simulink model "M4B11_modified_AGC_RL"  (R2025a)
settings: Solver=VariableStepAuto  StartTime=0.0  StopTime=100  RelTol=1e-3
InitFcn:
  | clear;
  | load('parameterinit.mat');
  | set_param('M4B11_modified_AGC_RL/Python2Sim1','value','[0 0]');
  | acom=100;
  | bcom=50;
  | lam=100;
  | rng('shuffle'); % 可选：先打乱 MATLAB 全局 RNG（不是必需，但说明意图）
  | seed1 = randi([1,2147483647]); % 生成 1 到 2^31-1 之间的整数
  | seed2 = randi([1,2147483647]);
values from neighbouring files (symbols this model uses):
  ACgirdinit =     [datainit.mat]    (also in parameterinit.mat)
  AVm0 = [11.3576294988 11.3576294988]    [datainit.mat]    (also in parameterinit.mat)
  commun = [1 1 1 0]    [datainit.mat]    (also in initAll.m = [1,1,1,0]; parameterinit.mat)
  DataDelay = [0  0; 0  0; 0  0; 0  0]    [datainit.mat]    (also in initAll.m = 0.0*DataDelay; parameterinit.mat)
  ESinit =     [datainit.mat]    (also in parameterinit.mat)
  fB = 50    [datainit.mat]    (also in initAll.m; parameterinit.mat)
  Geninit =     [datainit.mat]    (also in initAll.m = Generator_init(opdata,SynMach_in_gidx); parameterinit.mat)
  SgridB = 100    [datainit.mat]    (also in initAll.m = resultsac.baseMVA; parameterinit.mat)
  wB = 314.159265359    [datainit.mat]    (also in initAll.m; parameterinit.mat)
  Windinit =     [datainit.mat]    (also in parameterinit.mat)
undefined symbols (not defined in the file or in its folder): c1, c2, c3, c4, c5, c6, cp_nom, lambda_nom, P_wind_base, Pelec_base, Pnom
libraries: spsBistableLib x9, slpidlib x2, simulink_extras x2
(part 1 of 6)
settings Model: Creator=LinSiQi  LastModifiedBy=86182
settings SolverCC: AlgebraicLoopSolver=TrustRegion
settings DataIOCC: DSMLogging=off  ReturnWorkspaceOutputs=off  SignalLoggingName=logout
settings DebuggingCC: UnconnectedInputMsg=warning  UnconnectedOutputMsg=warning  UnconnectedLineMsg=warning  ArithmeticOperatorsInVariantConditions=warning
settings ModelReferenceCC: EnableRefExpFcnMdlSchedulingChecks=on
settings SFSimCC: CustomCodeUndefinedFunction=UseInterfaceOnly
settings RTWCC: GPUComputeCapability=3.5  DLArmComputeVersion=19.05
settings CodeAppCC: StateflowObjectComments=on
settings SimscapeCC: SimscapeNormalizeSystem=off

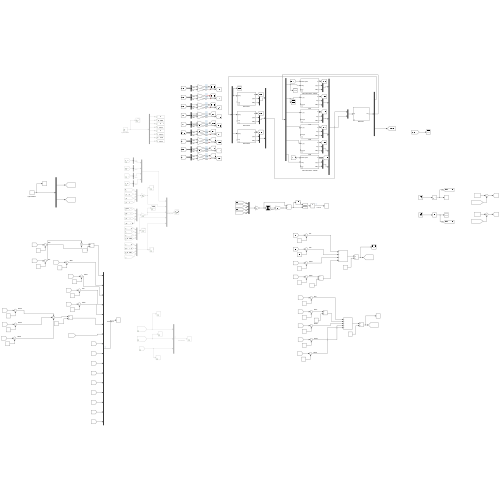
[thumbnail: Simulink's stored preview of the top-level diagram]
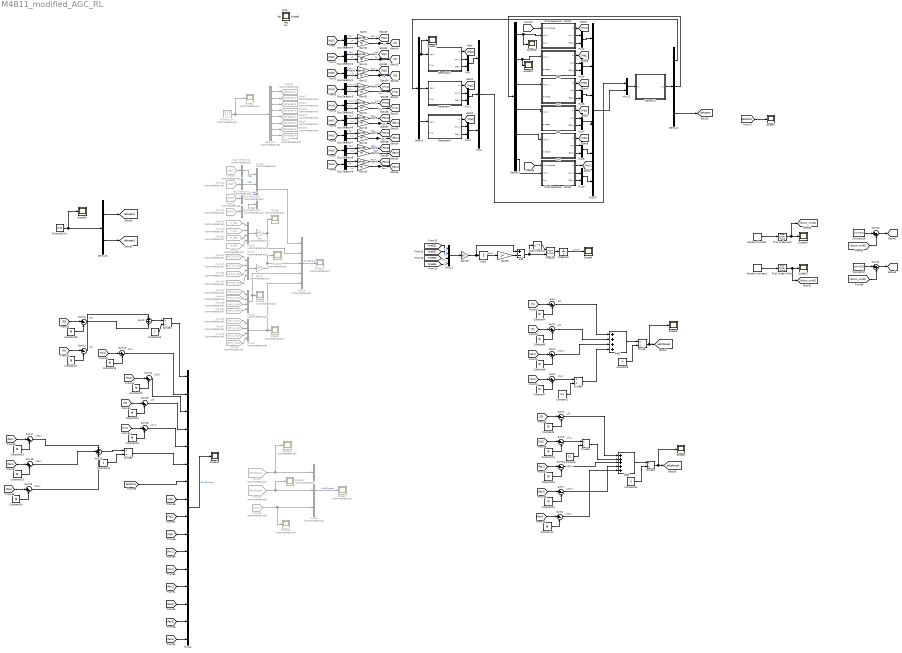
== system M4B11_modified_AGC_RL ==
  note: Δfes2
  note: Δfw2
  note: Δf3
  note: Δf1
  note: Δfes1
  note: Δfw1
  note: Δfes4
  note: Δf2
  note: Δfes3
  note: Δf1
  note: Δf2
  note: Δfw1
  note: Δfes1
  note: Δf3
  note: Δfw2
  note: Δfes4
  note: Δfes3
  note: Δfes2
  Add : Sum  Inputs=+-
  Add1 : Sum  Inputs=++++
  Add2 : Sum  Inputs=+
  Add3 : Sum  Inputs=+++++
  Bus Selector1 : BusSelector  OutputSignals=Pe,f
  Bus Selector{10..13} (4 alike) : BusSelector  Commented=on  OutputSignals=Pe
  Bus Selector2 : BusSelector  OutputSignals=Pe,f
  Bus Selector3 : BusSelector  OutputSignals=Pwind,fw
  Bus Selector4 : BusSelector  OutputSignals=Pe,f
  Bus Selector5 : BusSelector  OutputSignals=Pwind,fw
  Bus Selector{6..9} (4 alike) : BusSelector  OutputSignals=Pe,w
  Constant{4..7,9..10,12,15..25} (18 alike) : Constant  Value=fB
  Constant11 : Constant  Value=5
  Constant13 : Constant  Value=2
  Constant14 : Constant  Value=3
  Constant2 : Constant  Value=0.2
  Constant26 : Constant  Value=AVm0(1)
  Constant27 : Constant  Value=AVm0(2)
  Constant3 : Constant  Value=0.2
  Constant8 : Constant  Value=4
  Demux : Demux  Outputs=3
  Demux1 : Demux  Outputs=6
  Demux2 : Demux  Outputs=[6 12 1]
  Demux3 : Demux  Commented=on  Outputs=8
  Demux5 : Demux  Outputs=2
  Divide{,1..5} (6 alike) : Product  Inputs=*/
  ES1 : Subsystem  mask{SvscB=ESinit.SvscBi(1), SgridB=SgridB, Kppll_VSC=ESinit.Kppll(1), Kipll_VSC=ESinit.Kipll(1), Dels_hvdc=ESinit.Dels_hvdc(1), Lpr=ESinit.Lpr(1), Rpr=ESinit.Rpr(1), wB=wB, Is_xA_0=ESinit.Isx0(1), Is_yA_0=ESinit.Isy0(1), KpP_VSC_A=ESinit.KpP(1), KiP_VSC_A=ESinit.KiP(1), KpId_VSC_A=ESinit.KpId(1), KiId_VSC_A=ESinit.KiId(1), KpQ_VSC_A=ESinit.KpQ(1), KiQ_VSC_A=ESinit.KiQ(1), KpIq_VSC_A=ESinit.KpIq(1), KiIq_VSC_A=ESinit.KiIq(1), Md_A_0=ESinit.Md0(1), Mq_A_0=ESinit.Mq0(1), Nd_A_0=ESinit.Nd0(1), Nq_A_0=ESinit.Nq0(1), KIR=ESinit.Kir(1), Kdroop=ESinit.Kdroop(1), Kdistributed=ESinit.Kdistributed(1), Kdistributed_d=ESinit.Kdistributed_d(1), Kpac_VSC_A=ESinit.Kpac(1), Kiac_VSC_A=ESinit.Kiac(1), P0=ESinit.P0(1), Q0=ESinit.Q0(1), usd0=ESinit.Usd0(1)}
      mask prompts: Kppll_VSC "Kppll"; Kipll_VSC "Kipll"; KpP_VSC_A "KpP"; KiP_VSC_A "KiP"; KpId_VSC_A "KpId"; KiId_VSC_A "KiId"; KpQ_VSC_A "KpQ"; KiQ_VSC_A "KiQ"; KpIq_VSC_A "KpIq"; KiIq_VSC_A "KiIq"; Kpac_VSC_A "Kpac"; Kiac_VSC_A "Kiac"
      mask DialogControl Container48 Prompt: Base value
      mask DialogControl Container7 Prompt: PLL
      mask DialogControl Container5 Prompt: Control parameter
      mask DialogControl Container8 Prompt: inital value
      mask DialogControl Container9 Prompt: AC side
      mask DialogControl Container10 Prompt: Parameter
      mask DialogControl Container11 Prompt: Initial value
      mask DialogControl Container18 Prompt: Control parameter
      mask DialogControl Container19 Prompt: d_axis_control parameter
      mask DialogControl Container23 Prompt: d_axis_control=1
      mask DialogControl Container26 Prompt: inner current control
      mask DialogControl Container21 Prompt: q_axis_control parameter
      mask DialogControl Container29 Prompt: q_axis_control=1
      mask DialogControl Container31 Prompt: inner current control
      mask DialogControl Container22 Prompt: inital value
      mask DialogControl Container35 Prompt: outer controller
      mask DialogControl Container36 Prompt: inner control
      mask DialogControl Container27 Prompt: Inertia control
      mask DialogControl Container28 Prompt: droop control
      mask DialogControl Container300 Prompt: distributed control
      mask DialogControl Container301 Prompt: Droop distributed control
      mask DialogControl Container40 Prompt: usdq_control
      mask DialogControl Container41 Prompt: PQinitial
      mask DialogControl Container42 Prompt: usd0initial
  ES2 : Subsystem  mask{SvscB=ESinit.SvscBi(2), SgridB=SgridB, Kppll_VSC=ESinit.Kppll(2), Kipll_VSC=ESinit.Kipll(2), Dels_hvdc=ESinit.Dels_hvdc(2), Lpr=ESinit.Lpr(2), Rpr=ESinit.Rpr(2), wB=wB, Is_xA_0=ESinit.Isx0(2), Is_yA_0=ESinit.Isy0(2), KpP_VSC_A=ESinit.KpP(2), KiP_VSC_A=ESinit.KiP(2), KpId_VSC_A=ESinit.KpId(2), KiId_VSC_A=ESinit.KiId(2), KpQ_VSC_A=ESinit.KpQ(2), KiQ_VSC_A=ESinit.KiQ(2), KpIq_VSC_A=ESinit.KpIq(2), KiIq_VSC_A=ESinit.KiIq(2), Md_A_0=ESinit.Md0(2), Mq_A_0=ESinit.Mq0(2), Nd_A_0=ESinit.Nd0(2), Nq_A_0=ESinit.Nq0(2), KIR=ESinit.Kir(2), Kdroop=ESinit.Kdroop(2), Kdistributed=ESinit.Kdistributed(2), Kdistributed_d=ESinit.Kdistributed_d(2), Kpac_VSC_A=ESinit.Kpac(2), Kiac_VSC_A=ESinit.Kiac(2), P0=ESinit.P0(2), Q0=ESinit.Q0(2), usd0=ESinit.Usd0(2)}
      mask prompts: Kppll_VSC "Kppll"; Kipll_VSC "Kipll"; KpP_VSC_A "KpP"; KiP_VSC_A "KiP"; KpId_VSC_A "KpId"; KiId_VSC_A "KiId"; KpQ_VSC_A "KpQ"; KiQ_VSC_A "KiQ"; KpIq_VSC_A "KpIq"; KiIq_VSC_A "KiIq"; Kpac_VSC_A "Kpac"; Kiac_VSC_A "Kiac"
      mask DialogControl Container48 Prompt: Base value
      mask DialogControl Container7 Prompt: PLL
      mask DialogControl Container5 Prompt: Control parameter
      mask DialogControl Container8 Prompt: inital value
      mask DialogControl Container9 Prompt: AC side
      mask DialogControl Container10 Prompt: Parameter
      mask DialogControl Container11 Prompt: Initial value
      mask DialogControl Container18 Prompt: Control parameter
      mask DialogControl Container19 Prompt: d_axis_control parameter
      mask DialogControl Container23 Prompt: d_axis_control=1
      mask DialogControl Container26 Prompt: inner current control
      mask DialogControl Container21 Prompt: q_axis_control parameter
      mask DialogControl Container29 Prompt: q_axis_control=1
      mask DialogControl Container31 Prompt: inner current control
      mask DialogControl Container22 Prompt: inital value
      mask DialogControl Container35 Prompt: outer controller
      mask DialogControl Container36 Prompt: inner control
      mask DialogControl Container27 Prompt: Inertia control
      mask DialogControl Container28 Prompt: droop control
      mask DialogControl Container300 Prompt: distributed control
      mask DialogControl Container301 Prompt: Droop distributed control
      mask DialogControl Container40 Prompt: usdq_control
      mask DialogControl Container41 Prompt: PQinitial
      mask DialogControl Container42 Prompt: usd0initial
  ES3 : Subsystem  mask{SvscB=ESinit.SvscBi(3), SgridB=SgridB, Kppll_VSC=ESinit.Kppll(3), Kipll_VSC=ESinit.Kipll(3), Dels_hvdc=ESinit.Dels_hvdc(3), Lpr=ESinit.Lpr(3), Rpr=ESinit.Rpr(3), wB=wB, Is_xA_0=ESinit.Isx0(3), Is_yA_0=ESinit.Isy0(3), KpP_VSC_A=ESinit.KpP(3), KiP_VSC_A=ESinit.KiP(3), KpId_VSC_A=ESinit.KpId(3), KiId_VSC_A=ESinit.KiId(3), KpQ_VSC_A=ESinit.KpQ(3), KiQ_VSC_A=ESinit.KiQ(3), KpIq_VSC_A=ESinit.KpIq(3), KiIq_VSC_A=ESinit.KiIq(3), Md_A_0=ESinit.Md0(3), Mq_A_0=ESinit.Mq0(3), Nd_A_0=ESinit.Nd0(3), Nq_A_0=ESinit.Nq0(3), KIR=ESinit.Kir(3), Kdroop=ESinit.Kdroop(3), Kdistributed=ESinit.Kdistributed(3), Kdistributed_d=ESinit.Kdistributed_d(3), Kpac_VSC_A=ESinit.Kpac(3), Kiac_VSC_A=ESinit.Kiac(3), P0=ESinit.P0(3), Q0=ESinit.Q0(3), usd0=ESinit.Usd0(3)}
      mask prompts: Kppll_VSC "Kppll"; Kipll_VSC "Kipll"; KpP_VSC_A "KpP"; KiP_VSC_A "KiP"; KpId_VSC_A "KpId"; KiId_VSC_A "KiId"; KpQ_VSC_A "KpQ"; KiQ_VSC_A "KiQ"; KpIq_VSC_A "KpIq"; KiIq_VSC_A "KiIq"; Kpac_VSC_A "Kpac"; Kiac_VSC_A "Kiac"
      mask DialogControl Container48 Prompt: Base value
      mask DialogControl Container7 Prompt: PLL
      mask DialogControl Container5 Prompt: Control parameter
      mask DialogControl Container8 Prompt: inital value
      mask DialogControl Container9 Prompt: AC side
      mask DialogControl Container10 Prompt: Parameter
      mask DialogControl Container11 Prompt: Initial value
      mask DialogControl Container18 Prompt: Control parameter
      mask DialogControl Container19 Prompt: d_axis_control parameter
      mask DialogControl Container23 Prompt: d_axis_control=1
      mask DialogControl Container26 Prompt: inner current control
      mask DialogControl Container21 Prompt: q_axis_control parameter
      mask DialogControl Container29 Prompt: q_axis_control=1
      mask DialogControl Container31 Prompt: inner current control
      mask DialogControl Container22 Prompt: inital value
      mask DialogControl Container35 Prompt: outer controller
      mask DialogControl Container36 Prompt: inner control
      mask DialogControl Container27 Prompt: Inertia control
      mask DialogControl Container28 Prompt: droop control
      mask DialogControl Container300 Prompt: distributed control
      mask DialogControl Container301 Prompt: Droop distributed control
      mask DialogControl Container40 Prompt: usdq_control
      mask DialogControl Container41 Prompt: PQinitial
      mask DialogControl Container42 Prompt: usd0initial
  ES4 : Subsystem  mask{SvscB=ESinit.SvscBi(4), SgridB=SgridB, Kppll_VSC=ESinit.Kppll(4), Kipll_VSC=ESinit.Kipll(4), Dels_hvdc=ESinit.Dels_hvdc(4), Lpr=ESinit.Lpr(4), Rpr=ESinit.Rpr(4), wB=wB, Is_xA_0=ESinit.Isx0(4), Is_yA_0=ESinit.Isy0(4), KpP_VSC_A=ESinit.KpP(4), KiP_VSC_A=ESinit.KiP(4), KpId_VSC_A=ESinit.KpId(4), KiId_VSC_A=ESinit.KiId(4), KpQ_VSC_A=ESinit.KpQ(4), KiQ_VSC_A=ESinit.KiQ(4), KpIq_VSC_A=ESinit.KpIq(4), KiIq_VSC_A=ESinit.KiIq(4), Md_A_0=ESinit.Md0(4), Mq_A_0=ESinit.Mq0(4), Nd_A_0=ESinit.Nd0(4), Nq_A_0=ESinit.Nq0(4), KIR=ESinit.Kir(4), Kdroop=ESinit.Kdroop(4), Kdistributed=ESinit.Kdistributed(4), Kdistributed_d=ESinit.Kdistributed_d(4), Kpac_VSC_A=ESinit.Kpac(4), Kiac_VSC_A=ESinit.Kiac(4), P0=ESinit.P0(4), Q0=ESinit.Q0(4), usd0=ESinit.Usd0(4)}
      mask prompts: Kppll_VSC "Kppll"; Kipll_VSC "Kipll"; KpP_VSC_A "KpP"; KiP_VSC_A "KiP"; KpId_VSC_A "KpId"; KiId_VSC_A "KiId"; KpQ_VSC_A "KpQ"; KiQ_VSC_A "KiQ"; KpIq_VSC_A "KpIq"; KiIq_VSC_A "KiIq"; Kpac_VSC_A "Kpac"; Kiac_VSC_A "Kiac"
      mask DialogControl Container48 Prompt: Base value
      mask DialogControl Container7 Prompt: PLL
      mask DialogControl Container5 Prompt: Control parameter
      mask DialogControl Container8 Prompt: inital value
      mask DialogControl Container9 Prompt: AC side
      mask DialogControl Container10 Prompt: Parameter
      mask DialogControl Container11 Prompt: Initial value
      mask DialogControl Container18 Prompt: Control parameter
      mask DialogControl Container19 Prompt: d_axis_control parameter
      mask DialogControl Container23 Prompt: d_axis_control=1
      mask DialogControl Container26 Prompt: inner current control
      mask DialogControl Container21 Prompt: q_axis_control parameter
      mask DialogControl Container29 Prompt: q_axis_control=1
      mask DialogControl Container31 Prompt: inner current control
      mask DialogControl Container22 Prompt: inital value
      mask DialogControl Container35 Prompt: outer controller
      mask DialogControl Container36 Prompt: inner control
      mask DialogControl Container27 Prompt: Inertia control
      mask DialogControl Container28 Prompt: droop control
      mask DialogControl Container300 Prompt: distributed control
      mask DialogControl Container301 Prompt: Droop distributed control
      mask DialogControl Container40 Prompt: usdq_control
      mask DialogControl Container41 Prompt: PQinitial
      mask DialogControl Container42 Prompt: usd0initial
  First Order Hold : FirstOrderHold  ErrorTolerance=inf
  First Order Hold1 : FirstOrderHold  ErrorTolerance=inf
  From10 : From  Commented=on  GotoTag=Me2
  From11 : From  Commented=on  GotoTag=Me3
  From12 : From  Commented=on  GotoTag=Me4
  From27 : From  Commented=on  GotoTag=deltafarea1  TagVisibility=global
  From28 : From  Commented=on  GotoTag=deltafarea2  TagVisibility=global
  From29 : From  Commented=on  GotoTag=Ptie  TagVisibility=global
  From35 : From  Commented=on  GotoTag=Dess_avg4  TagVisibility=global
  From36 : From  Commented=on  GotoTag=Dess_avg3  TagVisibility=global
  From37 : From  Commented=on  GotoTag=Dess_avg2  TagVisibility=global
  From38 : From  Commented=on  GotoTag=Dess_avg1  TagVisibility=global
  From39 : From  Commented=on  GotoTag=Hess_avg3  TagVisibility=global
  From40 : From  Commented=on  GotoTag=Hess_avg2  TagVisibility=global
  From41 : From  Commented=on  GotoTag=Hess_avg1  TagVisibility=global
  From42 : From  Commented=on  GotoTag=W_ES1  TagVisibility=global
  From43 : From  Commented=on  GotoTag=ROCOF_ES1  TagVisibility=global
  From45 : From  Commented=on  GotoTag=Hess_avg4  TagVisibility=global
  From49 : From  Commented=on  GotoTag=W_ES2  TagVisibility=global
  From50 : From  Commented=on  GotoTag=ROCOF_ES2  TagVisibility=global
  From51 : From  Commented=on  GotoTag=W_ES3  TagVisibility=global
  From52 : From  Commented=on  GotoTag=ROCOF_ES3  TagVisibility=global
  From53 : From  Commented=on  GotoTag=W_ES4  TagVisibility=global
  From54 : From  Commented=on  GotoTag=ROCOF_ES4  TagVisibility=global
  From9 : From  Commented=on  GotoTag=Me1
  Gain : Gain  Commented=on  Gain=400
  Gain{1..9} (9 alike) : Gain  Gain=SgridB
  Gain{10..16,20..21} (9 alike) : Gain  Gain=fB
  Gain17 : Gain  Commented=on  Gain=200
  Gain18 : Gain  Gain=1/4
  Gain19 : Gain  Gain=50
  Generator1 : Subsystem  mask{wB=wB, SgenB=Geninit.SgenB(1), SgridB=SgridB, Xq=Geninit.Xq(1), Xq1=Geninit.Xq1(1), Xq11=Geninit.Xq11(1), Tq0=Geninit.Tq0(1), Tq10=Geninit.Tq10(1), Eq10=Geninit.Eq1(1), Eq110=Geninit.Eq11(1), Xd=Geninit.Xd(1), Xd1=Geninit.Xd1(1), Xd11=Geninit.Xd11(1), Td0=Geninit.Td0(1), Td10=Geninit.Td10(1), Ed10=Geninit.Ed1(1), Ed110=Geninit.Ed11(1), H=Geninit.Tj(1), D=Geninit.D(1), delta0=Geninit.Delta(1), w0=1, Pm0=Geninit.Pm0(1), Ka=Geninit.Ka(1), Tb=Geninit.Tb(1), Tc=Geninit.Tc(1), Efmin=Geninit.Efmin(1), Efmax=Geninit.Efmax(1), Vref=Geninit.Vref(1), Ef10=Geninit.Vf1(1), S_PSS=Geninit.EnablePSS(1), Kpss=Geninit.kpss(1), Tw_P=Geninit.Tw_P(1), T1_P=Geninit.T1_P(1), T2_P=Geninit.T2_P(1), T3_P=Geninit.T3_P(1), T4_P=Geninit.T4_P(1), Upmax=Geninit.Upmax(1), Upmin=Geninit.Upmin(1), S_Gov=Geninit.Enablegov(1), R=Geninit.R_G(1), Ts_G=Geninit.Ts_G(1), Tc_G=Geninit.Tc_G(1), T3_G=Geninit.T3_G(1), T4_G=Geninit.T4_G(1), T5_G=Geninit.T5_G(1), dPmax=Geninit.dPmax(1), dPmin=Geninit.dPmin(1)}
      mask prompts: S_PSS "Enable PSS"; Tw_P "Tw"; T1_P "T1"; T2_P "T2"; T3_P "T3"; T4_P "T4"; S_Gov "Enable Governor"; Ts_G "Ts"; Tc_G "Tc"; T3_G "T3"; T4_G "T4"; T5_G "T5"
      mask help: This is a six-order synchronous generator with exciter system, governor and PSS.
      mask DialogControl Container6 Prompt: Machine parameter
      mask DialogControl Container25 Prompt: Base value
      mask DialogControl Container3 Prompt: q axis parameter
      mask DialogControl ParameterGroupVar Prompt: d axis parameter
      mask DialogControl Container4 Prompt: machine parameter
      mask DialogControl Container12 Prompt: Excitation System parameter
      mask DialogControl Container22 Prompt: parameter
      mask DialogControl Container23 Prompt: inital value
      mask DialogControl Container10 Prompt: PSS parameter
      mask DialogControl Container13 Prompt: Governor parameter
  Generator2 : Subsystem  mask{wB=wB, SgenB=Geninit.SgenB(2), SgridB=SgridB, Xq=Geninit.Xq(2), Xq1=Geninit.Xq1(2), Xq11=Geninit.Xq11(2), Tq0=Geninit.Tq0(2), Tq10=Geninit.Tq10(2), Eq10=Geninit.Eq1(2), Eq110=Geninit.Eq11(2), Xd=Geninit.Xd(2), Xd1=Geninit.Xd1(2), Xd11=Geninit.Xd11(2), Td0=Geninit.Td0(2), Td10=Geninit.Td10(2), Ed10=Geninit.Ed1(2), Ed110=Geninit.Ed11(2), H=Geninit.Tj(2), D=Geninit.D(2), delta0=Geninit.Delta(2), w0=1, Pm0=Geninit.Pm0(2), Ka=Geninit.Ka(2), Tb=Geninit.Tb(2), Tc=Geninit.Tc(2), Efmin=Geninit.Efmin(2), Efmax=Geninit.Efmax(2), Vref=Geninit.Vref(2), Ef10=Geninit.Vf1(2), S_PSS=Geninit.EnablePSS(2), Kpss=Geninit.kpss(2), Tw_P=Geninit.Tw_P(2), T1_P=Geninit.T1_P(2), T2_P=Geninit.T2_P(2), T3_P=Geninit.T3_P(2), T4_P=Geninit.T4_P(2), Upmax=Geninit.Upmax(2), Upmin=Geninit.Upmin(2), S_Gov=Geninit.Enablegov(2), R=Geninit.R_G(2), Ts_G=Geninit.Ts_G(2), Tc_G=Geninit.Tc_G(2), T3_G=Geninit.T3_G(2), T4_G=Geninit.T4_G(2), T5_G=Geninit.T5_G(2), dPmax=Geninit.dPmax(2), dPmin=Geninit.dPmin(2)}
      mask prompts: S_PSS "Enable PSS"; Tw_P "Tw"; T1_P "T1"; T2_P "T2"; T3_P "T3"; T4_P "T4"; S_Gov "Enable Governor"; Ts_G "Ts"; Tc_G "Tc"; T3_G "T3"; T4_G "T4"; T5_G "T5"
      mask help: This is a six-order synchronous generator with exciter system, governor and PSS.
      mask DialogControl Container6 Prompt: Machine parameter
      mask DialogControl Container25 Prompt: Base value
      mask DialogControl Container3 Prompt: q axis parameter
      mask DialogControl ParameterGroupVar Prompt: d axis parameter
      mask DialogControl Container4 Prompt: machine parameter
      mask DialogControl Container12 Prompt: Excitation System parameter
      mask DialogControl Container22 Prompt: parameter
      mask DialogControl Container23 Prompt: inital value
      mask DialogControl Container10 Prompt: PSS parameter
      mask DialogControl Container13 Prompt: Governor parameter
  Generator3 : Subsystem  mask{wB=wB, SgenB=Geninit.SgenB(3), SgridB=SgridB, Xq=Geninit.Xq(3), Xq1=Geninit.Xq1(3), Xq11=Geninit.Xq11(3), Tq0=Geninit.Tq0(3), Tq10=Geninit.Tq10(3), Eq10=Geninit.Eq1(3), Eq110=Geninit.Eq11(3), Xd=Geninit.Xd(3), Xd1=Geninit.Xd1(3), Xd11=Geninit.Xd11(3), Td0=Geninit.Td0(3), Td10=Geninit.Td10(3), Ed10=Geninit.Ed1(3), Ed110=Geninit.Ed11(3), H=Geninit.Tj(3), D=Geninit.D(3), delta0=Geninit.Delta(3), w0=1, Pm0=Geninit.Pm0(3), Ka=Geninit.Ka(3), Tb=Geninit.Tb(3), Tc=Geninit.Tc(3), Efmin=Geninit.Efmin(3), Efmax=Geninit.Efmax(3), Vref=Geninit.Vref(3), Ef10=Geninit.Vf1(3), S_PSS=Geninit.EnablePSS(3), Kpss=Geninit.kpss(3), Tw_P=Geninit.Tw_P(3), T1_P=Geninit.T1_P(3), T2_P=Geninit.T2_P(3), T3_P=Geninit.T3_P(3), T4_P=Geninit.T4_P(3), Upmax=Geninit.Upmax(3), Upmin=Geninit.Upmin(3), S_Gov=Geninit.Enablegov(3), R=Geninit.R_G(3), Ts_G=Geninit.Ts_G(3), Tc_G=Geninit.Tc_G(3), T3_G=Geninit.T3_G(3), T4_G=Geninit.T4_G(3), T5_G=Geninit.T5_G(3), dPmax=Geninit.dPmax(3), dPmin=Geninit.dPmin(3)}
      mask prompts: S_PSS "Enable PSS"; Tw_P "Tw"; T1_P "T1"; T2_P "T2"; T3_P "T3"; T4_P "T4"; S_Gov "Enable Governor"; Ts_G "Ts"; Tc_G "Tc"; T3_G "T3"; T4_G "T4"; T5_G "T5"
      mask help: This is a six-order synchronous generator with exciter system, governor and PSS.
      mask DialogControl Container6 Prompt: Machine parameter
      mask DialogControl Container25 Prompt: Base value
      mask DialogControl Container3 Prompt: q axis parameter
      mask DialogControl ParameterGroupVar Prompt: d axis parameter
      mask DialogControl Container4 Prompt: machine parameter
      mask DialogControl Container12 Prompt: Excitation System parameter
      mask DialogControl Container22 Prompt: parameter
      mask DialogControl Container23 Prompt: inital value
      mask DialogControl Container10 Prompt: PSS parameter
      mask DialogControl Container13 Prompt: Governor parameter
  Goto10 : Goto  Commented=on  GotoTag=deltaDess1  TagVisibility=global
  Goto11 : Goto  Commented=on  GotoTag=deltaHess2  TagVisibility=global
  Goto12 : Goto  Commented=on  GotoTag=deltaHess1  TagVisibility=global
  Goto16 : Goto  Commented=on  GotoTag=deltaHess4  TagVisibility=global
  Goto17 : Goto  Commented=on  GotoTag=deltaHess3  TagVisibility=global
  Goto18 : Goto  Commented=on  GotoTag=deltaDess4  TagVisibility=global
  Goto19 : Goto  Commented=on  GotoTag=deltaDess3  TagVisibility=global
  Goto9 : Goto  Commented=on  GotoTag=deltaDess2  TagVisibility=global
  Integrator : Integrator
  Math Function : Math  Operator=transpose
  Mux{,1..3,5..9,11} (10 alike) : Mux  Inputs=2
  Mux10 : Mux  Inputs=6
  Mux{12,20..23} (5 alike) : Mux  Commented=on
  Mux13 : Mux
  Mux14 : Mux  Inputs=16
  Mux19 : Mux  Commented=on  Inputs=3
  Mux24 : Mux  Commented=on  Inputs=5
  Mux4 : Mux  Inputs=3
  Network1 : Subsystem  mask{busdata=ACgirdinit.busdata{1}, linedata=ACgirdinit.linedata{1}, VSS0=ACgirdinit.VSS0{1}, LINE=ACgirdinit.fline{1}, fbus=ACgirdinit.FBUS(1), ng=ACgirdinit.ng{1}, Currentin_idx=ACgirdinit.Currentin_idx{1}, amp=ACgirdinit.amp}
  Product : Product  Multiplication=Matrix(*)
  Python2Sim : Constant  Commented=on  Value=[0 0 0 0 0 0 0 0]
  Python2Sim1 : Constant  Value=[0 0]
  Random Number : RandomNumber  Variance=0  Seed=seed1  SampleTime=0.2
  Random Number1 : RandomNumber  Variance=0  Seed=seed2  SampleTime=0.2
  Scope{,1..4,10..12,14,16} (10 alike) : Scope  Commented=on
      Scope settings: ActiveDisplayYMinimum=-0.00781  ActiveDisplayYMaximum=0.06976  DataLoggingVariableName=ScopeData7
      Scope1 settings: ActiveDisplayYMinimum=-1  ActiveDisplayYMaximum=1  DataLoggingVariableName=ScopeData5
      Scope10 settings: ActiveDisplayYMinimum=-0.00781  ActiveDisplayYMaximum=0.06976
      Scope11 settings: ActiveDisplayYMinimum=-0.65989  ActiveDisplayYMaximum=0.16966  DataLoggingVariableName=ScopeData2
      Scope12 settings: ActiveDisplayYMinimum=-2.31076  ActiveDisplayYMaximum=1.65079  DataLoggingVariableName=ScopeData3
      Scope14 settings: ActiveDisplayYMinimum=-1  ActiveDisplayYMaximum=1  DataLoggingVariableName=ScopeData5
      Scope16 settings: ActiveDisplayYMinimum=-0.65989  ActiveDisplayYMaximum=0.16966  DataLoggingVariableName=ScopeData11
      Scope2 settings: ActiveDisplayYMinimum=-2.31076  ActiveDisplayYMaximum=1.65079  DataLoggingVariableName=ScopeData8
      Scope3 settings: ActiveDisplayYMinimum=-0.04265  ActiveDisplayYMaximum=0.38387  DataLoggingVariableName=ScopeData9
      Scope4 settings: ActiveDisplayYMinimum=-1  ActiveDisplayYMaximum=1  DataLoggingVariableName=ScopeData10
  Scope{5..9,13,15,17..21} (12 alike) : Scope
      Scope13 settings: ActiveDisplayYMinimum=-20.35289  ActiveDisplayYMaximum=182.95724
      Scope15 settings: ActiveDisplayYMinimum=-1  ActiveDisplayYMaximum=1
      Scope17 settings: DataLoggingVariableName=ScopeData16
      Scope18 settings: DataLoggingVariableName=ScopeData17
      Scope19 settings: ActiveDisplayYMinimum=-1  ActiveDisplayYMaximum=1  DataLoggingVariableName=ScopeData23
      Scope20 settings: ActiveDisplayYMinimum=-2.2489543876139111  ActiveDisplayYMaximum=3.3539392148111777  DataLoggingVariableName=ScopeData18
      Scope21 settings: ActiveDisplayYMinimum=-3.4452863653493173  ActiveDisplayYMaximum=3.6369803120359561  DataLoggingVariableName=ScopeData19
      Scope5 settings: ActiveDisplayYMinimum=-6E-10  ActiveDisplayYMaximum=5.2E-9
      Scope7 settings: ActiveDisplayYMinimum=-0.37863  ActiveDisplayYMaximum=3.18886  DataLoggingVariableName=ScopeData2
      Scope8 settings: ActiveDisplayYMinimum=-1.41249  ActiveDisplayYMaximum=12.71242  DataLoggingVariableName=ScopeData2
      Scope9 settings: ActiveDisplayYMinimum=-1.97687  ActiveDisplayYMaximum=17.79187  DataLoggingVariableName=ScopeData3
      Scope6 settings: ActiveDisplayYMinimum=49.70428094700177  ActiveDisplayYMaximum=50.075704699720347
  Sum{,1..8,11..19} (18 alike) : Sum  Inputs=|+-
  Sum10 : Sum  Inputs=+++
  Sum20 : Sum  Inputs=|++
  Sum21 : Sum  Inputs=|++
  Sum9 : Sum
  Wind Generator - DFIG1 : Subsystem  mask{NN=Windinit.NN(1), SwgBi=Windinit.SwgBi(1), SmecBi=100, SgridB=SgridB, Atheta=Windinit.Atheta(1), Kppll=Windinit.Kppll_wind(1), Kipll=Windinit.Kipll_wind(1), pitch=[500 45 2], Srotors=1.3, H=Windinit.H(1), Wr0=Windinit.Wr0(1), Xa=Windinit.Xa(1), Xa1=Windinit.Xa1(1), Lm=Windinit.Lm(1), Lr=Windinit.Lr(1), Rs=Windinit.Rs(1), Ls=Windinit.Ls(1), Ta0=Windinit.Ta0(1), NPf=Windinit.NPf(1), Za=Windinit.Za{1}, Ex0=Windinit.Ex_ref(1), Ey0=Windinit.Ey_ref(1), wB=wB, KpP_rw=Windinit.KpP_rw(1), KiP_rw=Windinit.KiP_rw(1), KpId_rw=Windinit.KpId_rw(1), KiId_rw=Windinit.KiId_rw(1), KpQ_rw=Windinit.KpQ_rw(1), KiQ_rw=Windinit.KiQ_rw(1), KpIq_rw=Windinit.KpIq_rw(1), KiIq_rw=Windinit.KiIq_rw(1), Ird_ref=Windinit.Ird_ref(1), Irq_ref=Windinit.Irq_ref(1), Qs0=Windinit.Qs0(1), KpDC_gw=Windinit.KpDC_gw(1), KiDC_gw=Windinit.KiDC_gw(1), KpId_gw=Windinit.KpId_gw(1), KiId_gw=Windinit.KiId_gw(1), KpIq_gw=Windinit.KpIq_gw(1), KiIq_gw=Windinit.KiIq_gw(1), Vdc_w=Windinit.Vdc_w(1), Icd_ref=Windinit.Icd_ref(1), Icq_ref=Windinit.Icq_ref(1), Vcd_ref=Windinit.Vcd_ref(1), Vcq_ref=Windinit.Vcq_ref(1), Lg=Windinit.Lg(1), Rg=Windinit.Rg(1), Icx0=Windinit.Icx0(1), Icy0=Windinit.Icy0(1), C_w=Windinit.C_w(1), Vdc0=Windinit.Vdc0(1)}
      mask prompts: pitch "pitch_gain，pitch_max，pitch_rate"; Srotors "Start Rotor Speed"; Ex0 "Ex"; Ey0 "Ey"
      mask init:
      | pitch_gain=pitch(1);
      | pitch_max=pitch(2);
      | pitch_rate=pitch(3);
      | 
      | %该风机模型的基准容量
      | 
      | SwgeqB=SwgBi.*NN;
      mask DialogControl Container4 Prompt: PLL/Wind turbine
      mask DialogControl Container31 Prompt: Base value
      mask DialogControl Container23 Prompt: PLL
      mask DialogControl Container6 Prompt: inital value
      mask DialogControl Container5 Prompt: PI parameter
      mask DialogControl Container24 Prompt: Wind turbine
      mask DialogControl Container25 Prompt: pitch control
      mask DialogControl Container7 Prompt: Machine parameter
      mask DialogControl Container8 Prompt: Rotor
      mask DialogControl Container9 Prompt: Machine
      mask DialogControl Container10 Prompt: parameter
      mask DialogControl Container11 Prompt: inital value
      mask DialogControl Container12 Prompt: Rotor side control
      mask DialogControl Container13 Prompt: Control parameter
      mask DialogControl Container14 Prompt: Initial value
      mask DialogControl Container15 Prompt: reactive power
      mask DialogControl Container16 Prompt: Grid side control
      mask DialogControl Container17 Prompt: parameter
      mask DialogControl Container18 Prompt: reference
      mask DialogControl Container19 Prompt: inital value
      mask DialogControl Container20 Prompt: converter function
      mask DialogControl Container21 Prompt: inital value
      mask DialogControl Container22 Prompt: DC function
  Wind Generator - DFIG2 : Subsystem  mask{NN=Windinit.NN(2), SwgBi=Windinit.SwgBi(2), SmecBi=100, SgridB=SgridB, Atheta=Windinit.Atheta(2), Kppll=Windinit.Kppll_wind(2), Kipll=Windinit.Kipll_wind(2), pitch=[500 45 2], Srotors=1.3, H=Windinit.H(2), Wr0=Windinit.Wr0(2), Xa=Windinit.Xa(2), Xa1=Windinit.Xa1(2), Lm=Windinit.Lm(2), Lr=Windinit.Lr(2), Rs=Windinit.Rs(2), Ls=Windinit.Ls(2), Ta0=Windinit.Ta0(2), NPf=Windinit.NPf(2), Za=Windinit.Za{2}, Ex0=Windinit.Ex_ref(2), Ey0=Windinit.Ey_ref(2), wB=wB, KpP_rw=Windinit.KpP_rw(2), KiP_rw=Windinit.KiP_rw(2), KpId_rw=Windinit.KpId_rw(2), KiId_rw=Windinit.KiId_rw(2), KpQ_rw=Windinit.KpQ_rw(2), KiQ_rw=Windinit.KiQ_rw(2), KpIq_rw=Windinit.KpIq_rw(2), KiIq_rw=Windinit.KiIq_rw(2), Ird_ref=Windinit.Ird_ref(2), Irq_ref=Windinit.Irq_ref(2), Qs0=Windinit.Qs0(2), KpDC_gw=Windinit.KpDC_gw(2), KiDC_gw=Windinit.KiDC_gw(2), KpId_gw=Windinit.KpId_gw(2), KiId_gw=Windinit.KiId_gw(2), KpIq_gw=Windinit.KpIq_gw(2), KiIq_gw=Windinit.KiIq_gw(2), Vdc_w=Windinit.Vdc_w(2), Icd_ref=Windinit.Icd_ref(2), Icq_ref=Windinit.Icq_ref(2), Vcd_ref=Windinit.Vcd_ref(2), Vcq_ref=Windinit.Vcq_ref(2), Lg=Windinit.Lg(2), Rg=Windinit.Rg(2), Icx0=Windinit.Icx0(2), Icy0=Windinit.Icy0(2), C_w=Windinit.C_w(2), Vdc0=Windinit.Vdc0(2)}
      mask prompts: pitch "pitch_gain，pitch_max，pitch_rate"; Srotors "Start Rotor Speed"; Ex0 "Ex"; Ey0 "Ey"
      mask init:
      | pitch_gain=pitch(1);
      | pitch_max=pitch(2);
      | pitch_rate=pitch(3);
      | 
      | %该风机模型的基准容量
      | 
      | SwgeqB=SwgBi.*NN;
      mask DialogControl Container4 Prompt: PLL/Wind turbine
      mask DialogControl Container31 Prompt: Base value
      mask DialogControl Container23 Prompt: PLL
      mask DialogControl Container6 Prompt: inital value
      mask DialogControl Container5 Prompt: PI parameter
      mask DialogControl Container24 Prompt: Wind turbine
      mask DialogControl Container25 Prompt: pitch control
      mask DialogControl Container7 Prompt: Machine parameter
      mask DialogControl Container8 Prompt: Rotor
      mask DialogControl Container9 Prompt: Machine
      mask DialogControl Container10 Prompt: parameter
      mask DialogControl Container11 Prompt: inital value
      mask DialogControl Container12 Prompt: Rotor side control
      mask DialogControl Container13 Prompt: Control parameter
      mask DialogControl Container14 Prompt: Initial value
      mask DialogControl Container15 Prompt: reactive power
      mask DialogControl Container16 Prompt: Grid side control
      mask DialogControl Container17 Prompt: parameter
      mask DialogControl Container18 Prompt: reference
      mask DialogControl Container19 Prompt: inital value
      mask DialogControl Container20 Prompt: converter function
      mask DialogControl Container21 Prompt: inital value
      mask DialogControl Container22 Prompt: DC function
  Pes : Scope
      settings: ActiveDisplayYMinimum=-12.906510922619532  ActiveDisplayYMaximum=250.25539940171976  DataLoggingVariableName=ScopeData4
  Pg : Scope
      settings: ActiveDisplayYMinimum=559.168910466539  ActiveDisplayYMaximum=845.17141516748893
  Pw : Scope
      settings: ActiveDisplayYMinimum=14.4539  ActiveDisplayYMaximum=655.57738  DataLoggingVariableName=ScopeData3
  fes : Scope
      settings: ActiveDisplayYMinimum=49.6543119958632  ActiveDisplayYMaximum=50.103977263973036  DataLoggingVariableName=ScopeData6
  fg : Scope
      settings: ActiveDisplayYMinimum=49.808347560980451  ActiveDisplayYMaximum=50.045408030054375  DataLoggingVariableName=ScopeData2
  tag scope: deltaPtie=global, deltafarea1=global, deltafarea2=global, deltapes1=global, deltapes3=global
  wires:
  Mux/1 -> Mux4/1
  Generator2/2(Igxy1) -> Mux1/1
  Generator3/2(Igxy1) -> Mux2/1
  Generator1/2(Igxy1) -> Mux/1
  Generator2/3(GBxy) -> Mux1/2
  Mux1/1 -> Mux4/2
  Mux2/1 -> Mux4/3
  Generator1/3(GBxy) -> Mux/2
  Generator3/3(GBxy) -> Mux2/2
  Demux/2 -> Generator2/1(Vgxy)
  Demux/3 -> Generator3/1(Vgxy)
  Demux1/1 -> Scope18/1, Wind Generator - DFIG1/2(Vsxy)
  Demux1/2 -> Scope19/1, ES1/1(us_xy)
  Demux1/3 -> ES2/1(us_xy)
  Demux1/4 -> ES3/1(us_xy)
  Demux1/5 -> ES4/1(us_xy)
  Demux1/6 -> Wind Generator - DFIG2/2(Vsxy)
  Wind Generator - DFIG1/3(GBxy) -> Mux3/2
  Mux3/1 -> Mux10/1
  Wind Generator - DFIG1/2(Igxy1) -> Mux3/1
  ES1/3(GBxy) -> Mux5/2
  Mux5/1 -> Mux10/2
  ES1/2(isxy) -> Mux5/1
  ES2/3(GBxy) -> Mux6/2
  Mux6/1 -> Mux10/3
  ES2/2(isxy) -> Mux6/1
  ES3/3(GBxy) -> Mux7/2
  Mux7/1 -> Mux10/4
  ES3/2(isxy) -> Mux7/1
  ES4/3(GBxy) -> Mux8/2
  Mux8/1 -> Mux10/5
  ES4/2(isxy) -> Mux8/1
  Wind Generator - DFIG2/3(GBxy) -> Mux9/2
  Mux9/1 -> Mux10/6
  Wind Generator - DFIG2/2(Igxy1) -> Mux9/1
  Network1/1(Vxy) -> Demux2/1
  Demux2/1 -> Demux/1
  Demux2/2 -> Demux1/1
  Mux11/1 -> Network1/1(Ixy)
  Mux4/1 -> Mux11/1
  Mux10/1 -> Mux11/2
  Generator1/1(m) -> [Mg1]
  Generator2/1(m) -> [Mg2]
  Generator3/1(m) -> [Mg3]
  Wind Generator - DFIG1/1(m) -> [Mw1]
  Wind Generator - DFIG2/1(m) -> [Mw2]
  ES2/1(m) -> [Me2]
  ES1/1(m) -> [Me1]
  ES3/1(m) -> [Me3]
  ES4/1(m) -> [Me4]
  [Mg1] -> Bus Selector4/1
  Bus Selector4/1 -> Gain6/1  "<Pe>"
  Bus Selector1/1 -> Gain1/1  "<Pe>"
  [Mg2] -> Bus Selector1/1
  Bus Selector1/2 -> Gain11/1  "<f>"
  Bus Selector2/1 -> Gain2/1  "<Pe>"
  [Mg3] -> Bus Selector2/1
  Bus Selector2/2 -> Gain12/1  "<f>"
  [Mw1] -> Bus Selector3/1
  Bus Selector3/1 -> Gain3/1  "<Pwind>"
  [Mw2] -> Bus Selector5/1
  Bus Selector5/1 -> Gain4/1  "<Pwind>"
  [Me1] -> Bus Selector6/1
  Bus Selector6/1 -> Gain5/1  "<Pe>"
  Gain6/1 -> [Pg1]  "Pg1"
  Gain1/1 -> ?  "Pg2"
  Gain2/1 -> [Pg3]  "Pg3"
  Gain3/1 -> [Pw1]  "Pw1"
  Gain4/1 -> [Pw2]  "Pw2"
  Gain5/1 -> [Pes1]  "Pes1"
  Gain7/1 -> [Pes2]  "Pes2"
  Bus Selector7/1 -> Gain7/1  "<Pe>"
  [Me2] -> Bus Selector7/1
  [Me3] -> Bus Selector8/1
  Bus Selector8/1 -> Gain8/1  "<Pe>"
  Gain8/1 -> [Pes3]  "Pes3"
  [Me4] -> Bus Selector9/1
  Bus Selector9/1 -> Gain9/1  "<Pe>"
  Gain9/1 -> [Pes4]  "Pes4"
  Gain10/1 -> [f1]  "f1"
  Bus Selector4/2 -> Gain10/1  "<f>"
  Gain11/1 -> [f2]  "f2"
  Gain12/1 -> [f3]  "f3"
  Demux3/4 -> Goto16/1
  Demux3/5 -> Goto10/1
  Demux3/6 -> Goto9/1
  Demux3/7 -> Goto19/1
  Python2Sim/1 -> Scope1/1, Demux3/1
  Demux3/2 -> Goto11/1
  Demux3/3 -> Goto17/1
  Demux3/1 -> Goto12/1
  Demux3/8 -> Goto18/1
  Bus Selector6/2 -> Gain13/1  "<w>"
  Bus Selector7/2 -> Gain14/1  "<w>"
  Bus Selector8/2 -> Gain15/1  "<w>"
  Bus Selector9/2 -> Gain16/1  "<w>"
  Gain13/1 -> [fes1]  "fes1"
  Gain14/1 -> [fes2]  "fes2"
  Gain15/1 -> [fes3]  "fes3"
  Gain16/1 -> [fes4]  "fes4"
  From9/1 -> Bus Selector10/1
  From10/1 -> Bus Selector11/1
  From11/1 -> Bus Selector12/1
  From12/1 -> Bus Selector13/1
  Bus Selector12/1 -> Mux12/3  "<Pe>"
  Bus Selector13/1 -> Mux12/4  "<Pe>"
  Bus Selector11/1 -> Mux12/2  "<Pe>"
  Bus Selector10/1 -> Mux12/1  "<Pe>"
  From42/1 -> Mux20/1
  From51/1 -> Mux20/3
  From53/1 -> Mux20/4
  From49/1 -> Mux20/2
  Gain/1 -> Scope/1, Mux24/2
  Mux20/1 -> Gain/1
  From52/1 -> Mux21/3
  From50/1 -> Mux21/2
  From54/1 -> Mux21/4
  From43/1 -> Mux21/1
  Gain17/1 -> Scope2/1, Mux24/3
  Mux21/1 -> Gain17/1
  Mux23/1 -> Mux24/4, Scope3/1
  From45/1 -> Mux23/4
  From40/1 -> Mux23/2
  From37/1 -> Mux22/2
  From35/1 -> Mux22/4
  From36/1 -> Mux22/3
  From39/1 -> Mux23/3
  From41/1 -> Mux23/1
  From38/1 -> Mux22/1
  Mux22/1 -> Mux24/5, Scope4/1
  Mux12/1 -> Mux24/1
  Mux24/1 -> Scope16/1  "Sim2Python"
  [WreES1] -> Mux13/1  "W1"
  [WreES2] -> Mux13/2  "W2"
  [WreES3] -> Mux13/3  "W3"
  [WreES4] -> Mux13/4  "W4"
  Gain19/1 -> Add/1, Add2/1
  Add2/1 -> Gain18/1  "Pess1"
  Gain18/1 -> Add/2
  Add/1 -> Product/2, Math Function/1
  Product/1 -> Integrator/1
  Integrator/1 -> Scope5/1  "L2norm"
  Math Function/1 -> Product/1
  Mux13/1 -> Gain19/1
  Demux2/3 -> [deltaPtie]
  Bus Selector3/2 -> Gain20/1  "<fw>"
  Bus Selector5/2 -> Gain21/1  "<fw>"
  Gain20/1 -> [fw1]  "fw1"
  Gain21/1 -> [fw2]  "fw2"
  [deltaPtie] -> Scope7/1
  Mux19/1 -> Scope11/1  "Sim2Python"
  From27/1 -> Scope10/1, Mux19/1
  From28/1 -> Scope12/1, Mux19/2
  From29/1 -> Scope14/1, Mux19/3
  Python2Sim1/1 -> Scope15/1, Demux5/1
  Demux5/2 -> [deltapes3]
  Demux5/1 -> [deltapes1]
  Mux14/1 -> Scope13/1  "Sim2Python"
  Sum9/1 -> Divide2/1
  Constant13/1 -> Divide2/2
  Constant14/1 -> Divide3/2
  Sum10/1 -> Divide3/1
  Divide2/1 -> Mux14/1
  Divide3/1 -> Mux14/6
  [deltaPtie] -> Mux14/7
  Divide5/1 -> Add3/2
  Sum8/1 -> Add3/5
  Divide4/1 -> Add1/4
  Sum4/1 -> Add3/1
  Constant8/1 -> Divide/2
  Add3/1 -> Divide1/1
  Constant5/1 -> Sum1/2
  Divide/1 -> Scope9/1, [deltafarea1]
  [fes3] -> Sum7/1
  [f1] -> Sum/1
  Constant7/1 -> Sum3/2
  Constant12/1 -> Sum8/2
  [fw1] -> Sum5/1
  Sum/1 -> Add1/1
  [fes4] -> Sum8/1
  Constant16/1 -> Sum6/2
  Add1/1 -> Divide/1
  [fes1] -> Sum2/1
  Sum5/1 -> Divide5/1
  Constant10/1 -> Sum7/2
  [f3] -> Sum4/1
  Sum6/1 -> Add3/3
  Constant15/1 -> Sum5/2
  Constant6/1 -> Sum2/2
  Constant11/1 -> Divide1/2
  [f2] -> Sum1/1
  Divide1/1 -> Scope8/1, [deltafarea2]
  Constant3/1 -> Divide5/2
  [fw2] -> Sum3/1
  Sum1/1 -> Add1/2
  Sum2/1 -> Add1/3
  Sum7/1 -> Add3/4
  Constant9/1 -> Sum4/2
  Constant4/1 -> Sum/2
  Constant2/1 -> Divide4/2
  Sum3/1 -> Divide4/1
  [fes2] -> Sum6/1
  Constant18/1 -> Sum12/2
  Sum12/1 -> Sum9/2
  [f1] -> Sum11/1
  [f2] -> Sum12/1
  Sum11/1 -> Sum9/1
  Constant17/1 -> Sum11/2
  Constant19/1 -> Sum13/2
  [fw2] -> Sum13/1
  Sum13/1 -> Mux14/2
  Constant20/1 -> Sum14/2
  [fes1] -> Sum14/1
  Sum14/1 -> Mux14/3
  [f3] -> Sum15/1
  Constant21/1 -> Sum15/2
  Sum15/1 -> Mux14/4
  Constant22/1 -> Sum16/2
  [fw1] -> Sum16/1
  Sum16/1 -> Mux14/5
  Sum19/1 -> Sum10/3
  Constant24/1 -> Sum19/2
  [fes3] -> Sum18/1
  Constant23/1 -> Sum18/2
  Sum17/1 -> Sum10/1
  Constant25/1 -> Sum17/2
  [fes4] -> Sum19/1
  Sum18/1 -> Sum10/2
  [fes2] -> Sum17/1
  [Pg1] -> Mux14/8
  [Pg2] -> Mux14/9
  [Pg3] -> Mux14/10
  [Pw1] -> Mux14/11
  [Pw2] -> Mux14/12
  [Pes1] -> Mux14/13
  [Pes2] -> Mux14/14
  [Pes3] -> Mux14/15
  [Pes4] -> Mux14/16
  Demux/1 -> Scope17/1, Generator1/1(Vgxy)
  Random Number/1 -> First Order Hold/1
  Random Number1/1 -> First Order Hold1/1
  First Order Hold/1 -> [distur_wind1], Scope20/1
  First Order Hold1/1 -> [distur_wind2], Scope21/1
  Constant26/1 -> Sum20/1
  [distur_wind1] -> Sum20/2
  Sum20/1 -> [AVm01]
  Sum21/1 -> [AVm02]
  Constant27/1 -> Sum21/1
  [distur_wind2] -> Sum21/2
  [AVm01] -> Wind Generator - DFIG1/1(Wind speed)
  [AVm02] -> Wind Generator - DFIG2/1(Wind speed)
